simulink model "gm_NexusA7MLmodel"  (R2024a)
settings: Solver=FixedStepDiscrete  StartTime=0.0  StopTime=80  FixedStep=1  RelTol=1e-3
undefined symbols (not defined in the file or in its folder): t0, t1, t2, t3, t4, t5, t6, t7
libraries: dspsrcs4 x8
settings Model: Creator=MonishKS  LastModifiedBy=user
settings OptimizationCC: BlockReduction=off  ConditionallyExecuteInputs=off  DefaultParameterBehavior=Inlined  InheritOutputTypeSmallerThanSingle=on
settings DebuggingCC: ArtificialAlgebraicLoopMsg=error  InheritedTsInSrcMsg=none  SingleTaskRateTransMsg=error
settings HardwareCC: ProdBitPerPointer=32  ProdBitPerSizeT=32  ProdBitPerPtrDiffT=32  ProdLargestAtomicFloat=None  ProdIntDivRoundTo=Undefined  ProdEndianess=Unspecified  ProdWordSize=32  ProdHWDeviceType=ASIC/FPGA->ASIC/FPGA  TargetBitPerPointer=64  TargetBitPerSizeT=64  TargetBitPerPtrDiffT=64  TargetLongLongMode=on  TargetIntDivRoundTo=Zero  TargetEndianess=LittleEndian  TargetWordSize=64  TargetHWDeviceType=Custom Processor->MATLAB Host Computer  ProdEqTarget=off

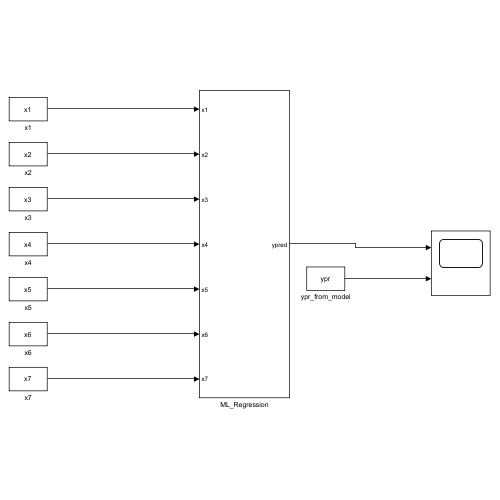
[thumbnail: Simulink's stored preview of the top-level diagram]
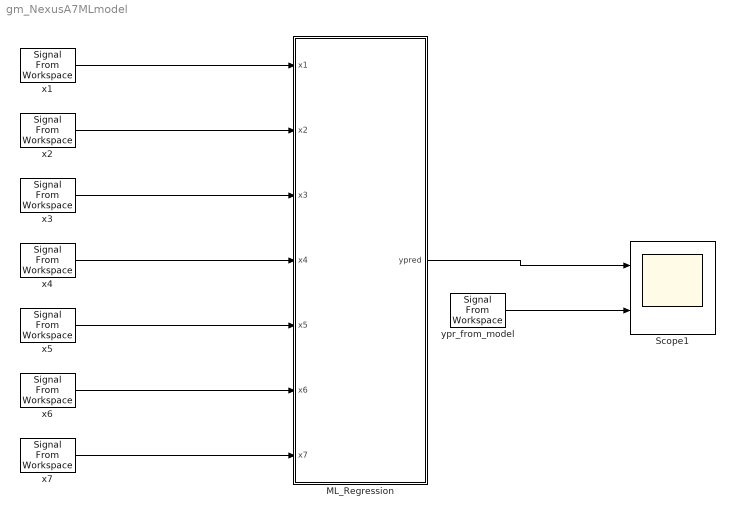
== system gm_NexusA7MLmodel ==
  ML_Regression : Subsystem
  Scope1 : Scope  NumInputPorts=2
  x1 : dspsrcs4/Signal From Workspace  X=x1  Ts=-1  nsamps=1  OutputAfterFinalValue=Setting to zero  ignoreOrWarnInputAndFrameLengths=off  OutputFrames=off
  x2 : dspsrcs4/Signal From Workspace  X=x2  Ts=-1  nsamps=1  OutputAfterFinalValue=Setting to zero  ignoreOrWarnInputAndFrameLengths=off  OutputFrames=off
  x3 : dspsrcs4/Signal From Workspace  X=x3  Ts=-1  nsamps=1  OutputAfterFinalValue=Setting to zero  ignoreOrWarnInputAndFrameLengths=off  OutputFrames=off
  x4 : dspsrcs4/Signal From Workspace  X=x4  Ts=-1  nsamps=1  OutputAfterFinalValue=Setting to zero  ignoreOrWarnInputAndFrameLengths=off  OutputFrames=off
  x5 : dspsrcs4/Signal From Workspace  X=x5  Ts=-1  nsamps=1  OutputAfterFinalValue=Setting to zero  ignoreOrWarnInputAndFrameLengths=off  OutputFrames=off
  x6 : dspsrcs4/Signal From Workspace  X=x6  Ts=-1  nsamps=1  OutputAfterFinalValue=Setting to zero  ignoreOrWarnInputAndFrameLengths=off  OutputFrames=off
  x7 : dspsrcs4/Signal From Workspace  X=x7  Ts=-1  nsamps=1  OutputAfterFinalValue=Setting to zero  ignoreOrWarnInputAndFrameLengths=off  OutputFrames=off
  ypr_from_model : dspsrcs4/Signal From Workspace  X=ypr  Ts=-1  nsamps=1  OutputAfterFinalValue=Setting to zero  ignoreOrWarnInputAndFrameLengths=off  OutputFrames=off
  wires:
  ML_Regression/1(ypred) -> Scope1/1
  ypr_from_model/1 -> Scope1/2
  x7/1 -> ML_Regression/7(x7)
  x6/1 -> ML_Regression/6(x6)
  x5/1 -> ML_Regression/5(x5)
  x4/1 -> ML_Regression/4(x4)
  x3/1 -> ML_Regression/3(x3)
  x2/1 -> ML_Regression/2(x2)
  x1/1 -> ML_Regression/1(x1)

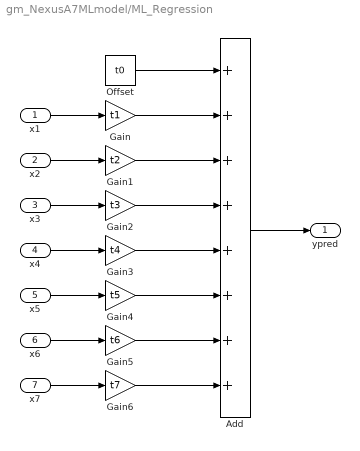
== system gm_NexusA7MLmodel/ML_Regression ==
  x1 : Inport
  x2 : Inport  Port=2
  x3 : Inport  Port=3
  x4 : Inport  Port=4
  x5 : Inport  Port=5
  x6 : Inport  Port=6
  x7 : Inport  Port=7
  Add : Sum  Inputs=++++++++  OutDataTypeStr=fixdt(0,16,16)
  Gain : Gain  Gain=t1
  Gain1 : Gain  Gain=t2
  Gain2 : Gain  Gain=t3
  Gain3 : Gain  Gain=t4
  Gain4 : Gain  Gain=t5
  Gain5 : Gain  Gain=t6
  Gain6 : Gain  Gain=t7
  Offset : Constant  Value=t0  OutDataTypeStr=fixdt(1,16,14)  SampleTime=-1
  ypred : Outport
  wires:
  Offset/1 -> Add/1
  Gain1/1 -> Add/3
  Gain/1 -> Add/2
  Gain4/1 -> Add/6
  Gain2/1 -> Add/4
  Add/1 -> ypred/1
  Gain3/1 -> Add/5
  x6/1 -> Gain5/1
  x5/1 -> Gain4/1
  Gain6/1 -> Add/8
  x7/1 -> Gain6/1
  x2/1 -> Gain1/1
  Gain5/1 -> Add/7
  x4/1 -> Gain3/1
  x1/1 -> Gain/1
  x3/1 -> Gain2/1
